simulink model "RefModel_FaultPanel"  (R2020a)
settings: Solver=ode1  StartTime=tspan(1)  StopTime=tspan(2)  FixedStep=Ts_SignalIntegrity.Ts_base  RelTol=1e-3
undefined symbols (not defined in the file or in its folder): airspeed1, baro1, ENUM_Fault, IMU1, IMU2, IMU3, mag1, mag2, radar1, ublox1, um482
settings Model: Creator=sl  LastModifiedBy=Administrator
settings SolverCC: AutoInsertRateTranBlk=on
settings DataIOCC: SaveOutput=off  SaveTime=off
settings OptimizationCC: DefaultParameterBehavior=Inlined  EnhancedBackFolding=on  PassReuseOutputArgsAs=Individual arguments  ZeroExternalMemoryAtStartup=off  ZeroInternalMemoryAtStartup=off  MaxStackSize=64  OptimizeBlockOrder=speed  DifferentSizesBufferReuse=on  OptimizationCustomize=off  EfficientTunableParamExpr=on
settings DebuggingCC: InheritedTsInSrcMsg=none  MultiTaskCondExecSysMsg=none  ParameterTunabilityLossMsg=error  UnconnectedInputMsg=none  UnconnectedOutputMsg=none  UnconnectedLineMsg=none  BusObjectLabelMismatch=error
settings HardwareCC: ProdBitPerPointer=32  ProdBitPerSizeT=32  ProdBitPerPtrDiffT=32  ProdLargestAtomicInteger=Long  ProdLargestAtomicFloat=Double  ProdWordSize=32  ProdHWDeviceType=ARM Compatible->ARM Cortex
settings ModelReferenceCC: EnableParallelModelReferenceBuilds=on  ParallelModelReferenceMATLABWorkerInit=Load Top Model
settings SFSimCC: MATLABDynamicMemAlloc=off
settings RTWCC: SystemTargetFile=ert.tlc  TemplateMakefile=ert_default_tmf  GenerateReport=on  Toolchain=GNU Tools for ARM Embedded Processors  IncludeHyperlinkInReport=on  LaunchReport=on  GenerateTraceInfo=on  GenerateTraceReport=on  GenerateTraceReportSl=on  GenerateTraceReportSf=on  GenerateTraceReportEml=on
settings CodeAppCC: ForceParamTrailComments=on  IgnoreCustomStorageClasses=off  OperatorAnnotations=on  SimulinkDataObjDesc=on  SFDataObjDesc=on  InsertBlockDesc=on
settings ERTTargetCC: InlinedParameterPlacement=NonHierarchical  ERTCustomFileTemplate=example_file_process.tlc

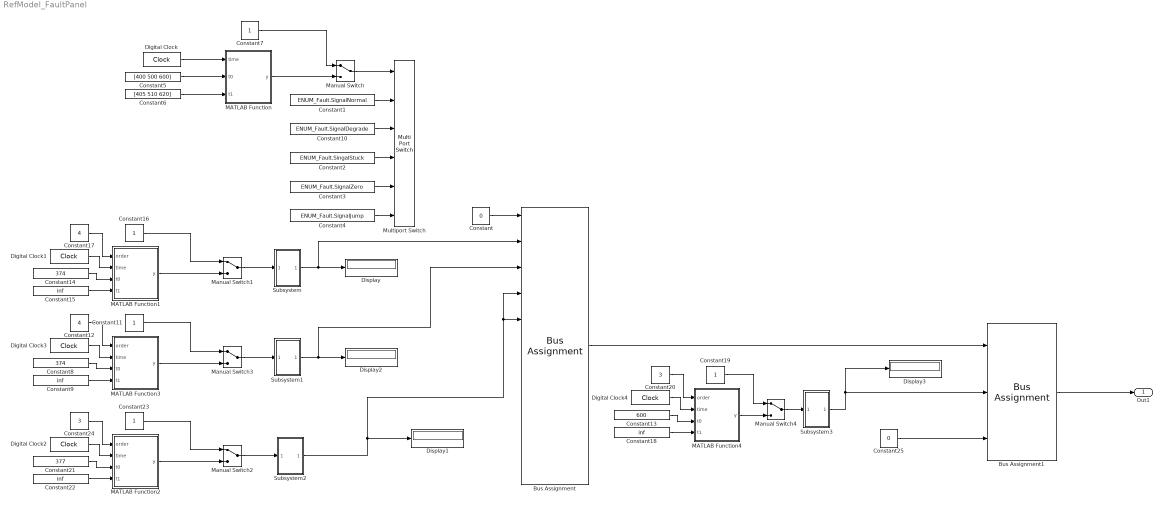
== system RefModel_FaultPanel ==
  Bus Assignment : BusAssignment  AssignedSignals=ublox1.status,um482.status,mag1.status,mag2.status,radar1.status,airspeed1.status,baro1.status,IMU1.status,IMU3.status,IMU2.status
  Bus Assignment1 : BusAssignment  AssignedSignals=airspeed1.status,airspeed1.offset1
  Constant : Constant  Value=0  OutDataTypeStr=Bus: BUS_SENSORFAULT_IN
  Constant1 : Constant  Value=ENUM_Fault.SignalNormal  OutDataTypeStr=Enum: ENUM_Fault
  Constant10 : Constant  Value=ENUM_Fault.SignalDegrade  OutDataTypeStr=Enum: ENUM_Fault
  Constant{7,11,16,19,23} (5 alike) : Constant
  Constant12 : Constant  Value=4
  Constant13 : Constant  Value=600
  Constant14 : Constant  Value=374
  Constant{9,15,18,22} (4 alike) : Constant  Value=inf
  Constant17 : Constant  Value=4
  Constant2 : Constant  Value=ENUM_Fault.SingalStuck  OutDataTypeStr=Enum: ENUM_Fault
  Constant20 : Constant  Value=3
  Constant21 : Constant  Value=377
  Constant24 : Constant  Value=3
  Constant25 : Constant  Value=0
  Constant3 : Constant  Value=ENUM_Fault.SignalZero  OutDataTypeStr=Enum: ENUM_Fault
  Constant4 : Constant  Value=ENUM_Fault.SignalJump  OutDataTypeStr=Enum: ENUM_Fault
  Constant5 : Constant  Value=[400 500 600]
  Constant6 : Constant  Value=[405 510 620]
  Constant8 : Constant  Value=374
  Digital Clock{,1..4} (5 alike) : DigitalClock  SampleTime=-1
  Display{,1..3} (4 alike) : Display
  MATLAB Function : MATLAB Function  TreatAsAtomicUnit=on
  MATLAB Function1 : MATLAB Function  TreatAsAtomicUnit=on
  MATLAB Function2 : MATLAB Function  TreatAsAtomicUnit=on
  MATLAB Function3 : MATLAB Function  TreatAsAtomicUnit=on
  MATLAB Function4 : MATLAB Function  TreatAsAtomicUnit=on
  Manual Switch{,1..4} (5 alike) : ManualSwitch
  Multiport Switch : MultiPortSwitch  Inputs=5
  Subsystem : Subsystem
  Subsystem1 : Subsystem
  Subsystem2 : Subsystem
  Subsystem3 : Subsystem
  Out1 : Outport  OutDataTypeStr=Bus: BUS_SENSORFAULT_IN  PortDimensions=1  BusOutputAsStruct=on
  wires:
  Constant4/1 -> Multiport Switch/6
  Constant3/1 -> Multiport Switch/5
  Constant10/1 -> Multiport Switch/3
  Constant2/1 -> Multiport Switch/4
  Constant1/1 -> Multiport Switch/2
  Constant/1 -> Bus Assignment/1
  Constant5/1 -> MATLAB Function/2(t0)
  Constant6/1 -> MATLAB Function/3(t1)
  Digital Clock/1 -> MATLAB Function/1(time)
  Manual Switch/1 -> Multiport Switch/1
  MATLAB Function/1(y) -> Manual Switch/2
  Constant7/1 -> Manual Switch/1
  Constant16/1 -> Manual Switch1/1
  MATLAB Function1/1(y) -> Manual Switch1/2
  Digital Clock1/1 -> MATLAB Function1/2(time)
  Constant15/1 -> MATLAB Function1/4(t1)
  Constant14/1 -> MATLAB Function1/3(t0)
  Constant17/1 -> MATLAB Function1/1(order)
  Constant24/1 -> MATLAB Function2/1(order)
  Constant21/1 -> MATLAB Function2/3(t0)
  Constant22/1 -> MATLAB Function2/4(t1)
  Digital Clock2/1 -> MATLAB Function2/2(time)
  MATLAB Function2/1(y) -> Manual Switch2/2
  Constant23/1 -> Manual Switch2/1
  Subsystem2/1(Out1) -> Display1/1, Bus Assignment/5, Bus Assignment/4
  Subsystem/1(Out1) -> Bus Assignment/2, Display/1
  Manual Switch1/1 -> Subsystem/1(In1)
  Manual Switch3/1 -> Subsystem1/1(In1)
  Subsystem1/1(Out1) -> Bus Assignment/3, Display2/1
  Constant12/1 -> MATLAB Function3/1(order)
  Constant8/1 -> MATLAB Function3/3(t0)
  Constant9/1 -> MATLAB Function3/4(t1)
  Digital Clock3/1 -> MATLAB Function3/2(time)
  MATLAB Function3/1(y) -> Manual Switch3/2
  Constant11/1 -> Manual Switch3/1
  Manual Switch2/1 -> Subsystem2/1(In1)
  Bus Assignment/1 -> Bus Assignment1/1
  Bus Assignment1/1 -> Out1/1
  Constant20/1 -> MATLAB Function4/1(order)
  Constant13/1 -> MATLAB Function4/3(t0)
  Constant19/1 -> Manual Switch4/1
  Subsystem3/1(Out1) -> Display3/1, Bus Assignment1/2
  MATLAB Function4/1(y) -> Manual Switch4/2
  Digital Clock4/1 -> MATLAB Function4/2(time)
  Manual Switch4/1 -> Subsystem3/1(In1)
  Constant18/1 -> MATLAB Function4/4(t1)
  Constant25/1 -> Bus Assignment1/3

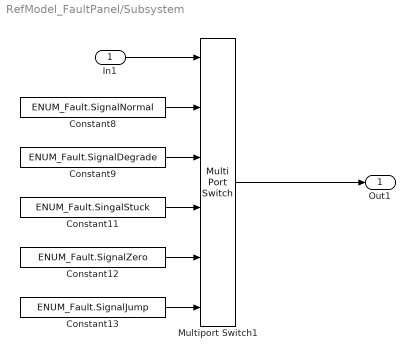
== system RefModel_FaultPanel/Subsystem ==
  In1 : Inport
  Constant11 : Constant  Value=ENUM_Fault.SingalStuck  OutDataTypeStr=Enum: ENUM_Fault
  Constant12 : Constant  Value=ENUM_Fault.SignalZero  OutDataTypeStr=Enum: ENUM_Fault
  Constant13 : Constant  Value=ENUM_Fault.SignalJump  OutDataTypeStr=Enum: ENUM_Fault
  Constant8 : Constant  Value=ENUM_Fault.SignalNormal  OutDataTypeStr=Enum: ENUM_Fault
  Constant9 : Constant  Value=ENUM_Fault.SignalDegrade  OutDataTypeStr=Enum: ENUM_Fault
  Multiport Switch1 : MultiPortSwitch  Inputs=5
  Out1 : Outport
  wires:
  Constant11/1 -> Multiport Switch1/4
  Constant8/1 -> Multiport Switch1/2
  In1/1 -> Multiport Switch1/1
  Constant13/1 -> Multiport Switch1/6
  Constant9/1 -> Multiport Switch1/3
  Constant12/1 -> Multiport Switch1/5
  Multiport Switch1/1 -> Out1/1

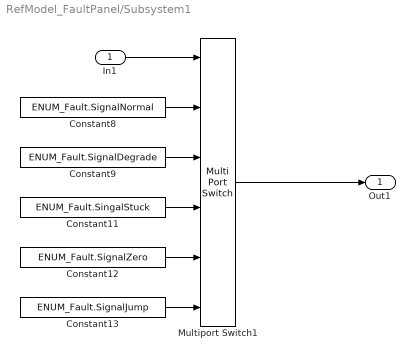
== system RefModel_FaultPanel/Subsystem1 ==
  In1 : Inport
  Constant11 : Constant  Value=ENUM_Fault.SingalStuck  OutDataTypeStr=Enum: ENUM_Fault
  Constant12 : Constant  Value=ENUM_Fault.SignalZero  OutDataTypeStr=Enum: ENUM_Fault
  Constant13 : Constant  Value=ENUM_Fault.SignalJump  OutDataTypeStr=Enum: ENUM_Fault
  Constant8 : Constant  Value=ENUM_Fault.SignalNormal  OutDataTypeStr=Enum: ENUM_Fault
  Constant9 : Constant  Value=ENUM_Fault.SignalDegrade  OutDataTypeStr=Enum: ENUM_Fault
  Multiport Switch1 : MultiPortSwitch  Inputs=5
  Out1 : Outport
  wires:
  Multiport Switch1/1 -> Out1/1
  Constant12/1 -> Multiport Switch1/5
  Constant9/1 -> Multiport Switch1/3
  Constant13/1 -> Multiport Switch1/6
  In1/1 -> Multiport Switch1/1
  Constant8/1 -> Multiport Switch1/2
  Constant11/1 -> Multiport Switch1/4

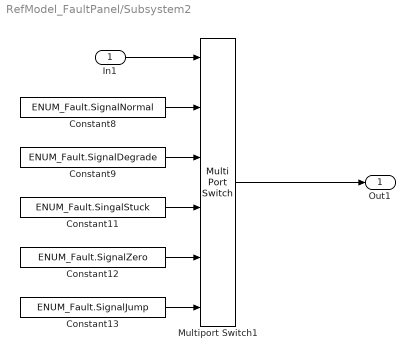
== system RefModel_FaultPanel/Subsystem2 ==
  In1 : Inport
  Constant11 : Constant  Value=ENUM_Fault.SingalStuck  OutDataTypeStr=Enum: ENUM_Fault
  Constant12 : Constant  Value=ENUM_Fault.SignalZero  OutDataTypeStr=Enum: ENUM_Fault
  Constant13 : Constant  Value=ENUM_Fault.SignalJump  OutDataTypeStr=Enum: ENUM_Fault
  Constant8 : Constant  Value=ENUM_Fault.SignalNormal  OutDataTypeStr=Enum: ENUM_Fault
  Constant9 : Constant  Value=ENUM_Fault.SignalDegrade  OutDataTypeStr=Enum: ENUM_Fault
  Multiport Switch1 : MultiPortSwitch  Inputs=5
  Out1 : Outport
  wires:
  Constant11/1 -> Multiport Switch1/4
  Constant8/1 -> Multiport Switch1/2
  In1/1 -> Multiport Switch1/1
  Constant13/1 -> Multiport Switch1/6
  Constant9/1 -> Multiport Switch1/3
  Constant12/1 -> Multiport Switch1/5
  Multiport Switch1/1 -> Out1/1

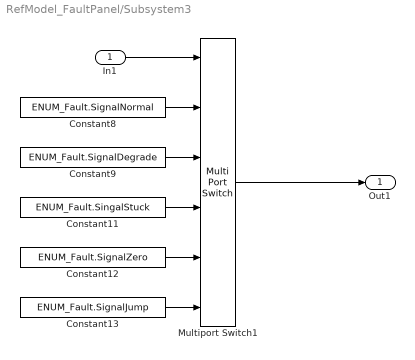
== system RefModel_FaultPanel/Subsystem3 ==
  In1 : Inport
  Constant11 : Constant  Value=ENUM_Fault.SingalStuck  OutDataTypeStr=Enum: ENUM_Fault
  Constant12 : Constant  Value=ENUM_Fault.SignalZero  OutDataTypeStr=Enum: ENUM_Fault
  Constant13 : Constant  Value=ENUM_Fault.SignalJump  OutDataTypeStr=Enum: ENUM_Fault
  Constant8 : Constant  Value=ENUM_Fault.SignalNormal  OutDataTypeStr=Enum: ENUM_Fault
  Constant9 : Constant  Value=ENUM_Fault.SignalDegrade  OutDataTypeStr=Enum: ENUM_Fault
  Multiport Switch1 : MultiPortSwitch  Inputs=5
  Out1 : Outport
  wires:
  Multiport Switch1/1 -> Out1/1
  Constant12/1 -> Multiport Switch1/5
  Constant9/1 -> Multiport Switch1/3
  Constant13/1 -> Multiport Switch1/6
  In1/1 -> Multiport Switch1/1
  Constant8/1 -> Multiport Switch1/2
  Constant11/1 -> Multiport Switch1/4

== matlab function RefModel_FaultPanel/MATLAB Function1 ==
  data: order input; time input; t0 input; y output; t1 input
function y = fcn(order, time, t0, t1)
% idx = 1;
y = 1;
for idx = 1:length(t0)
    if time > t0(idx) && time < t1(idx)
        y = order;
    end
end
% idx = 2;
% if time > t0(idx) && time < t1(idx)
%     y = order;
% end
% idx = 3;
% if time > t0(idx) && time < t1(idx)
%     y = order;
% end

== matlab function RefModel_FaultPanel/MATLAB Function ==
  data: time input; t0 input; y output; t1 input
function y = fcn(time, t0,t1)
idx = 1;
y = 1;
if time > t0(idx) && time < t1(idx)
    y = 2;
end
idx = 2;
if time > t0(idx) && time < t1(idx)
    y = 2;
end
idx = 3;
if time > t0(idx) && time < t1(idx)
    y = 2;
end

== matlab function RefModel_FaultPanel/MATLAB Function2 ==
  data: order input; time input; t0 input; y output; t1 input
function y = fcn(order, time, t0, t1)
% idx = 1;
y = 1;
for idx = 1:length(t0)
    if time > t0(idx) && time < t1(idx)
        y = order;
    end
end
% idx = 2;
% if time > t0(idx) && time < t1(idx)
%     y = order;
% end
% idx = 3;
% if time > t0(idx) && time < t1(idx)
%     y = order;
% end

== matlab function RefModel_FaultPanel/MATLAB Function3 ==
  data: order input; time input; t0 input; y output; t1 input
function y = fcn(order, time, t0, t1)
% idx = 1;
y = 1;
for idx = 1:length(t0)
    if time > t0(idx) && time < t1(idx)
        y = order;
    end
end
% idx = 2;
% if time > t0(idx) && time < t1(idx)
%     y = order;
% end
% idx = 3;
% if time > t0(idx) && time < t1(idx)
%     y = order;
% end

== matlab function RefModel_FaultPanel/MATLAB Function4 ==
  data: order input; time input; t0 input; y output; t1 input
function y = fcn(order, time, t0, t1)
% idx = 1;
y = 1;
for idx = 1:length(t0)
    if time > t0(idx) && time < t1(idx)
        y = order;
    end
end
% idx = 2;
% if time > t0(idx) && time < t1(idx)
%     y = order;
% end
% idx = 3;
% if time > t0(idx) && time < t1(idx)
%     y = order;
% end
